simulink model "Propeller"  (Simulink 8.3)
settings: Solver=ode45  StartTime=0.0  StopTime=10.0  RelTol=1e-3
settings Model: Creator=Administrator  LastModifiedBy=Administrator
settings DataIOCC: SignalLoggingSaveFormat=Dataset
settings DebuggingCC: UnderspecifiedInitializationDetection=Simplified  StateNameClashWarn=none
settings GRTTargetCC: CombineOutputUpdateFcns=on  GRTInterface=off

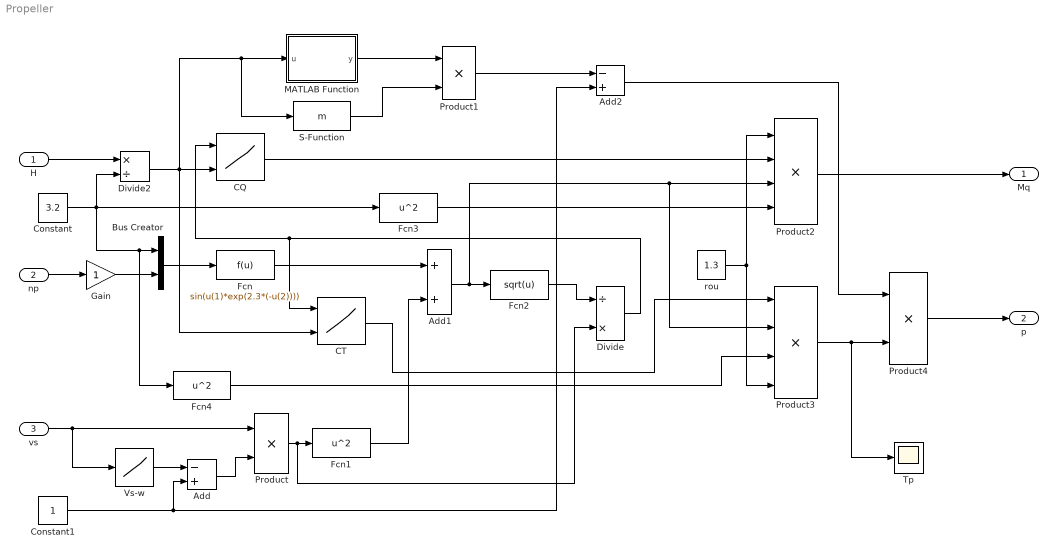
== system Propeller ==
  H : Inport
  np : Inport  Port=2
  vs : Inport  Port=3
  Add : Sum  Inputs=-+
  Add1 : Sum
  Add2 : Sum  Inputs=-+
  Bus Creator : BusCreator  Inputs=2
  CQ : Lookup_n-D  BreakpointsForDimension1=[1:3]  BreakpointsForDimension2=[1:3]  InternalRulePriority=Speed  RndMeth=Simplest  InputSameDT=on
  CT : Lookup_n-D  BreakpointsForDimension1=[1:3]  BreakpointsForDimension2=[1:3]  InternalRulePriority=Speed  RndMeth=Simplest  InputSameDT=on
  Constant : Constant  Value=3.2
  Constant1 : Constant
  Divide : Product  Inputs=/*
  Divide2 : Product  Inputs=*/
  Fcn : Fcn  Expr=sin(u(1)*exp(2.3*(-u(2))))
  Fcn1 : Fcn  Expr=u^2
  Fcn2 : Fcn  Expr=sqrt(u)
  Fcn3 : Fcn  Expr=u^2
  Fcn4 : Fcn  Expr=u^2
  Gain : Gain
  MATLAB Function : MATLAB Function  TreatAsAtomicUnit=on
  Product : Product
  Product1 : Product
  Product2 : Product  Inputs=4
  Product3 : Product  Inputs=4
  Product4 : Product
  S-Function : S-Function  FunctionName=m  EnableBusSupport=off
  Tp : Scope
  Vs-w : Lookup_n-D  NumberOfTableDimensions=1  BreakpointsForDimension1=[-5:5]  Table=tanh([-5:5])  InternalRulePriority=Speed  RndMeth=Simplest  InputSameDT=on
  rou : Constant  Value=1.3
  Mq : Outport
  p : Outport  Port=2
  wires:
  H/1 -> Divide2/1
  Divide2/1 -> CT/2, CQ/2, S-Function/1, MATLAB Function/1(u)
  MATLAB Function/1(y) -> Product1/1
  S-Function/1 -> Product1/2
  Product1/1 -> Add2/1
  Constant/1 -> Bus Creator/1, Fcn4/1, Fcn3/1, Divide2/2
  np/1 -> Gain/1
  Constant1/1 -> Add/2, Add2/2
  Add/1 -> Product/2
  Product/1 -> Divide/2, Fcn1/1
  Fcn1/1 -> Add1/2
  Gain/1 -> Bus Creator/2
  Bus Creator/1 -> Fcn/1
  Fcn3/1 -> Product2/4
  Fcn4/1 -> Product3/3
  Product3/1 -> Tp/1, Product4/2
  Add2/1 -> Product4/1
  Product2/1 -> Mq/1
  Product4/1 -> p/1
  rou/1 -> Product3/4, Product2/1
  Add1/1 -> Fcn2/1, Product3/2, Product2/3
  Fcn2/1 -> Divide/1
  Fcn/1 -> Add1/1
  vs/1 -> Vs-w/1, Product/1
  Vs-w/1 -> Add/1
  CQ/1 -> Product2/2
  Divide/1 -> CT/1, CQ/1
  CT/1 -> Product3/1

== matlab function MATLAB Function ==
  data: u input double; y output double
function y = fcn(u)
% This block supports the Embedded MATLAB subset.
% See the help menu for details. 

if u<=-1
    y=3
elseif u<=0
    y=(-3)*u
elseif u<1
    y=u
else
    y=1
end
